simulink subsystem "RackAndPinion"  (R2023a)
settings: Solver=VariableStepAuto  StartTime=0.0  StopTime=10.0  RelTol=1e-3
model mask{i_rp=20000, vis_friction_coef_rp=0.002, J_pinion=1e-6}
settings Model: Creator=mrrom  LastModifiedBy=romav

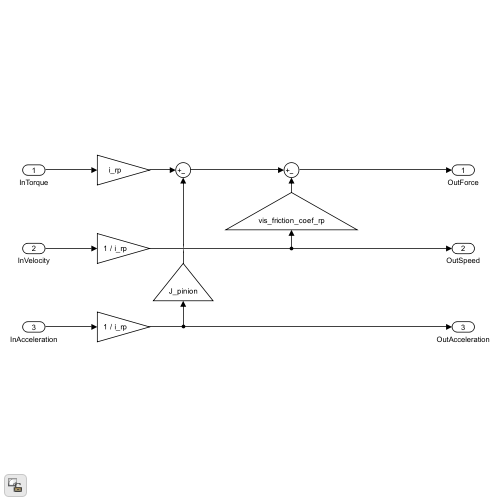
[thumbnail: Simulink's stored preview of the top-level diagram]
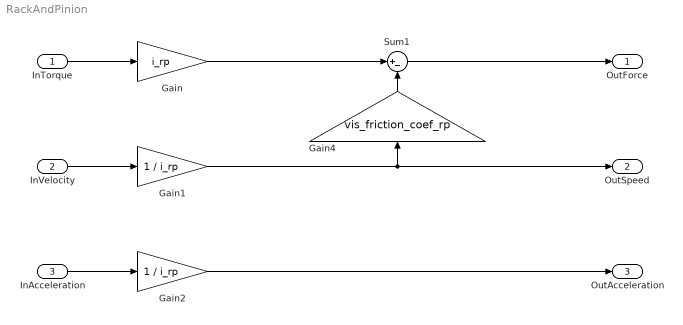
== system RackAndPinion ==
  InTorque : Inport
  InVelocity : Inport  Port=2
  InAcceleration : Inport  Port=3
  Gain : Gain  Gain=i_rp
  Gain1 : Gain  Gain=1 / i_rp
  Gain2 : Gain  Gain=1 / i_rp
  Gain4 : Gain  Gain=vis_friction_coef_rp
  Sum1 : Sum  Inputs=|+-
  OutForce : Outport
  OutSpeed : Outport  Port=2
  OutAcceleration : Outport  Port=3
  wires:
  Gain1/1 -> Gain4/1, OutSpeed/1
  Sum1/1 -> OutForce/1
  InVelocity/1 -> Gain1/1
  InTorque/1 -> Gain/1
  Gain/1 -> Sum1/1
  InAcceleration/1 -> Gain2/1
  Gain4/1 -> Sum1/2
  Gain2/1 -> OutAcceleration/1
